simulink model "Lift_Parallel_logic"  (R2020b)
settings: Solver=VariableStepAuto  StartTime=0.0  StopTime=10.0  RelTol=1e-3
settings Model: Creator=Manoj  LastModifiedBy=Windows 10

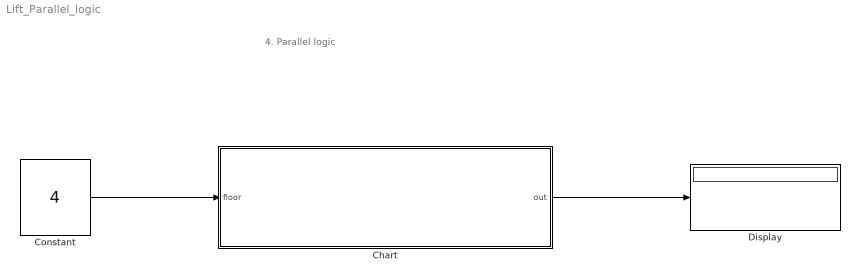
== system Lift_Parallel_logic ==
  note: 4. Parallel logic
  Chart : Stateflow chart  TreatAsAtomicUnit=on
  Constant : Constant  Value=4
  Display : Display
  wires:
  Constant/1 -> Chart/1(floor)
  Chart/1(out) -> Display/1

== stateflow chart Lift_Parallel_logic/Chart ==
  state active [parallel]
    settings: executionOrder=1
    state stop
      out=current;
    state up
      entry:
      current=0;
      du:
      current=current+1;
    state down
      entry:
      current=0;
      du:
      current=current-1;
    (default) -> stop : {current=1;}
    stop -> stop [order 1] : [floor==current]
    stop -> up [order 2] : [current<floor]
    stop -> down [order 3] : [current>floor]
    up -> stop [order 1] : [current==floor]
    down -> stop : [current==floor]
    up -> up [order 2] : [current<floor]
  state floor [parallel]
    settings: executionOrder=2
    state s2
      entry:
      out=2;
      current=out;
    state s1
      entry:
      current=1;
      out=1;
    state s3
      entry:
      out=3;
      current=out;
    state s4
      entry:
      out=4;
      current=out;
    state s5
      entry:
      out=5;
      current=out;
    s1 -> s1 [order 2] : [current==floor]
    (default) -> s1
    s1 -> s2 [order 1] : [current<floor]
    s4 -> s3 [order 2] : [current>floor]
    s2 -> s3 [order 1] : [current<floor]
    s2 -> s1 [order 2] : [current>floor]
    s3 -> s2 [order 2] : [current>floor]
    s3 -> s4 [order 1] : [current<floor]
    s5 -> s4 [order 1] : [current>floor]
    s4 -> s5 [order 1] : [current<floor]
    s5 -> s5 [order 2] : [floor==current]
  data: floor input; out output; current local
